simulink model "test_reference_signal"  (R2019b)
settings: Solver=VariableStepAuto  StartTime=0.0  StopTime=10.0  RelTol=1e-3
values from neighbouring files (symbols this model uses):
  Zc = 0.32    [Parameters_Init.m]    (also in test.m = 0.35)
libraries: powerlib_meascontrol x2
settings Model: Creator=wangcanye  LastModifiedBy=wangcanye

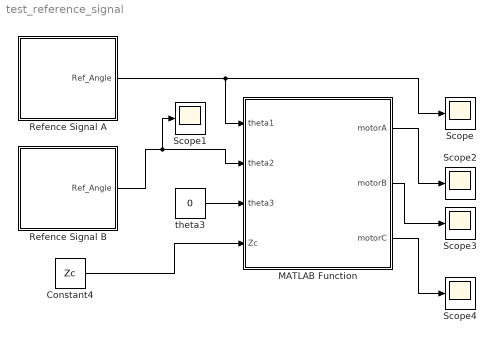
== system test_reference_signal ==
  Constant4 : Constant  Value=Zc
  MATLAB Function : MATLAB Function  TreatAsAtomicUnit=on
  Refence Signal A : Subsystem
  Refence Signal B : Subsystem
  Scope{,1..4} (5 alike) : Scope
  theta3 : Constant  Value=0
  wires:
  Refence Signal A/1(Ref_Angle) -> Scope/1, MATLAB Function/1(theta1)
  Refence Signal B/1(Ref_Angle) -> Scope1/1, MATLAB Function/2(theta2)
  theta3/1 -> MATLAB Function/3(theta3)
  Constant4/1 -> MATLAB Function/4(Zc)
  MATLAB Function/1(motorA) -> Scope2/1
  MATLAB Function/2(motorB) -> Scope3/1
  MATLAB Function/3(motorC) -> Scope4/1

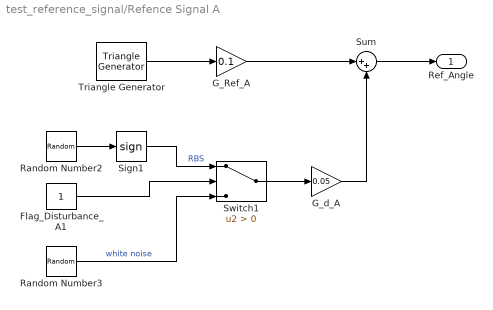
== system test_reference_signal/Refence Signal A ==
  Flag_Disturbance_A1 : Constant
  G_Ref_A : Gain  Gain=0.1
  G_d_A : Gain  Gain=0.05
  Random Number2 : RandomNumber  SampleTime=0.001
  Random Number3 : RandomNumber  SampleTime=0.001
  Sign1 : Signum
  Sum : Sum  Inputs=|++
  Switch1 : Switch  Criteria=u2 > Threshold
  Triangle Generator : powerlib_meascontrol/Pulse & Signal Generators/Triangle Generator  Freq=0.5  Phase=90  Ts=0
      settings: SourceProductName=Simscape Electrical
  Ref_Angle : Outport
  wires:
  Sign1/1 -> Switch1/1  "RBS"
  Switch1/1 -> G_d_A/1
  Random Number2/1 -> Sign1/1
  Triangle Generator/1 -> G_Ref_A/1
  Flag_Disturbance_A1/1 -> Switch1/2
  Random Number3/1 -> Switch1/3  "white noise"
  Sum/1 -> Ref_Angle/1
  G_Ref_A/1 -> Sum/1
  G_d_A/1 -> Sum/2

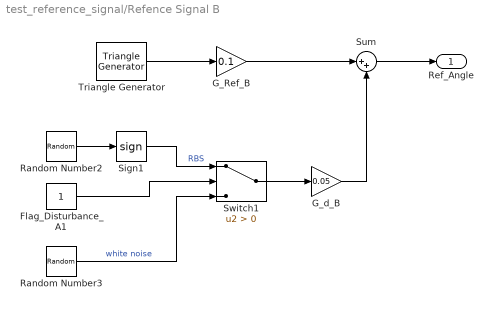
== system test_reference_signal/Refence Signal B ==
  Flag_Disturbance_A1 : Constant
  G_Ref_B : Gain  Gain=0.1
  G_d_B : Gain  Gain=0.05
  Random Number2 : RandomNumber  SampleTime=0.001
  Random Number3 : RandomNumber  SampleTime=0.001
  Sign1 : Signum
  Sum : Sum  Inputs=|++
  Switch1 : Switch  Criteria=u2 > Threshold
  Triangle Generator : powerlib_meascontrol/Pulse & Signal Generators/Triangle Generator  Freq=0.5  Phase=90  Ts=0
      settings: SourceProductName=Simscape Electrical
  Ref_Angle : Outport
  wires:
  Sign1/1 -> Switch1/1  "RBS"
  Switch1/1 -> G_d_B/1
  Random Number2/1 -> Sign1/1
  Triangle Generator/1 -> G_Ref_B/1
  Flag_Disturbance_A1/1 -> Switch1/2
  Random Number3/1 -> Switch1/3  "white noise"
  Sum/1 -> Ref_Angle/1
  G_Ref_B/1 -> Sum/1
  G_d_B/1 -> Sum/2

== matlab function test_reference_signal/MATLAB Function ==
  data: theta1 input; motorA output; theta2 input; theta3 input; Zc input; motorB output; motorC output
function [motorA, motorB, motorC] = anglesToMotors(theta1,theta2,theta3,Zc)

%% Define parameters
r = 0.17;
r0B1 = [r; 0; 0];      
r0B2 = [-0.5*r; (sqrt(3)/2)*r; 0];
r0B3 = [-0.5*r; -(sqrt(3)/2)*r; 0];
r0B = [r0B1 r0B2 r0B3];
%r1C1 = r0B1; r1C2 = r0B2; r1C3 = r0B3;
r1C = r0B;
r0Oc = [0;0;Zc];

% Find cos and sin to accelerate calculations
C1 = cos(theta1);S1 = sin(theta1);C2 = cos(theta2);S2 = sin(theta2);C3 = cos(theta3);S3 = sin(theta3);

% Rotation matrices
RotZ = [C3 S3 0; -S3 C3 0; 0 0 1];
RotY = [C2 0 -S2; 0 1 0; S2 0 C2];
RotX = [1 0 0; 0 C1 S1; 0 -S1 C1];

A10 = RotX*RotY*RotZ; A01 = A10';

% Find rCiBi (Vectors representing the motors)
rCiBi = zeros(3,3);
for i=1:3
    rCiBi(:,i) = r0Oc + A01*r1C(:,i) - r0B(:,i);
end

% Outputs to motor are the lengths of the vectors
motorA = norm(rCiBi(:,1));
motorB = norm(rCiBi(:,2));
motorC = norm(rCiBi(:,3));

end
